simulink model "spin"  (R2022b)
settings: Solver=VariableStepAuto  StartTime=0.0  StopTime=100  RelTol=1e-3
values from neighbouring files (symbols this model uses):
  delta = [0.5 1 1.5 2 2.5 3 3.5 4 4.5 5 5.5 6 ... (40 elements, 20x2)]    [delta.mat]
  v = [0.5 1 1.5 2 2.5 3 3.5 4 4.5 5 5.5 6 ... (40 elements, 20x2)]    [v.mat]
libraries: Solver_SF x1
settings Model: Creator=ASOAT  LastModifiedBy=ASOAT

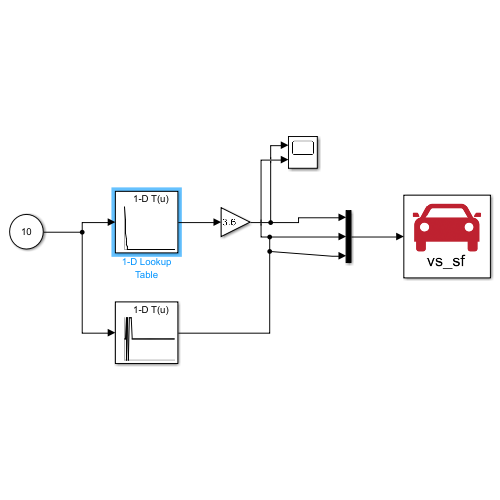
[thumbnail: Simulink's stored preview of the top-level diagram]
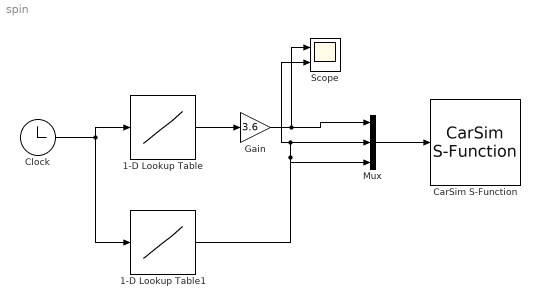
== system spin ==
  1-D Lookup Table : Lookup_n-D  NumberOfTableDimensions=1  BreakpointsForDimension1=v(1:120,1)  Table=v(1:120,2)  InternalRulePriority=Speed  RndMeth=Simplest
  1-D Lookup Table1 : Lookup_n-D  NumberOfTableDimensions=1  BreakpointsForDimension1=delta(1:64,1)  Table=delta(1:64,2)  InternalRulePriority=Speed  RndMeth=Simplest
  CarSim S-Function : Solver_SF/CarSim S-Function  Priority=1  SIMFILE=simfile.sim  Run_RTs=off  vs_state_ind=Run  StopMode_ind=Vehicle Model
  Clock : Clock
  Gain : Gain  Gain=3.6
  Mux : Mux  Inputs=3
  Scope : Scope  NumInputPorts=2
  wires:
  1-D Lookup Table1/1 -> Mux/3, Mux/2, Scope/2
  1-D Lookup Table/1 -> Gain/1
  Clock/1 -> 1-D Lookup Table/1, 1-D Lookup Table1/1
  Gain/1 -> Scope/1, Mux/1
  Mux/1 -> CarSim S-Function/1
